simulink library "xpcueilib"  (Simulink 6.0)
settings: Solver=ode45  SolverMode=SingleTasking  StartTime=0.0  StopTime=10.0  RelTol=1e-3
(part 1 of 2)
settings Model: Creator=adowd  LastModifiedBy=adowd
settings DataIOCC: SignalLoggingName=logsOut
settings OptimizationCC: BooleanDataType=off
settings DebuggingCC: CheckExecutionContextPreStartOutputMsg=on  CheckExecutionContextRuntimeOutputMsg=on  SolverPrmCheckMsg=none
settings HardwareCC: TargetUnknown=on
settings GRTTargetCC: UtilityFuncGeneration=Automatic  LifeSpan=inf
settings SFSimCC: SFSimApplyToAllLibs=on  SFSimBuildMode=Incremental

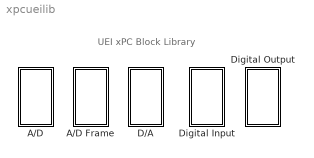
== system xpcueilib ==
  note: UEI xPC Block Library
  A/D : Subsystem  EnableExecutionContextPropagation=on
  A/D Frame : Subsystem  EnableExecutionContextPropagation=on
  D/A : Subsystem  EnableExecutionContextPropagation=on
  Digital Input : Subsystem  EnableExecutionContextPropagation=on
  Digital Output : Subsystem  EnableExecutionContextPropagation=on

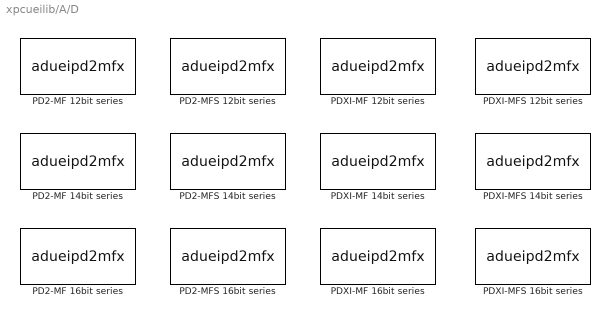
== system xpcueilib/A/D ==
  "PD2-MF 12bit series " : S-Function  InitFcn=muei  FunctionName=adueipd2mfx  Parameters=channel, gain, mux, range, sampletime, pcislot, boardType, gainval, board, devName  mask(ueipd2mf12_ad_7){boardtypein=PD2-MF-16-1M/12L, channel=[1], gain=[1], mux=[1], range=+- 10 Volts, sampletime=0.001, pcislot=-1}
      mask prompts: boardtypein "Board type:"; channel "Channel vector:"; gain "Gain vector:"; mux "Mux settling time vector (slow bit):"; pcislot "PCI slot (-1: autosearch):"
      mask help:
      | PD2-MF 12bit series
      | United Electronic Industries
      | Analog Input
      mask init:
      | [board, boardType, devName, gain, gainval, mux, maskdisplay, maskdescription]= madueipd2mfx(boardtypein,channel, gain, mux, pcislot);
      | set_param(gcb,'MaskDescription',maskdescription);
      | set_param(gcb,'MaskDisplay',maskdisplay);
      mask Help: helpview(fullfile(docroot, 'mapfiles', 'xpc.map'), 'UEI_PD2-MF-12bit-series_AD')
      mask StyleString: popup(PD2-MF-16-1M/12L|PD2-MF-16-1M/12H|PD2-MF-64-1M/12L|PD2-MF-64-1M/12H),edit,edit,edit,popup(+- 10 Volts|+- 5 Volts|0-10 Volts|0-5 Volts),edit,edit
      mask Display: disp('PD2-MF-16-1M/12L\nUEI\nAnalog Input');port_label('output',1,'1');
  "PD2-MF 14bit series " : S-Function  InitFcn=muei  FunctionName=adueipd2mfx  Parameters=channel, gain, mux, range, sampletime, pcislot, boardType, gainval, board, devName  mask(ueipd2mf14_ad_7){boardtypein=PD2-MF-16-400/14L, channel=[1], gain=[1], mux=[1], range=+- 10 Volts, sampletime=0.001, pcislot=-1}
      mask prompts: boardtypein "Board type:"; channel "Channel vector:"; gain "Gain vector:"; mux "Mux settling time vector (slow bit):"; pcislot "PCI slot (-1: autosearch):"
      mask help:
      | PD2-MF 14bit series
      | United Electronic Industries
      | Analog Input
      mask init: same as xpcueilib/A/D/PD2-MF 12bit series 
      mask Help: helpview(fullfile(docroot, 'mapfiles', 'xpc.map'), 'UEI_PD2-MF-14bit-series_AD')
      mask StyleString: popup(PD2-MF-16-400/14L|PD2-MF-16-400/14H|PD2-MF-64-400/14L|PD2-MF-64-400/14H|PD2-MF-16-800/14L|PD2-MF-16-800/14H|PD2-MF-64-800/14L|PD2-MF-64-800/14H|PD2-MF-16-2M/14L|PD2-MF-16-2M/14H|PD2-MF-64-2M/14L|PD2-MF-64-2M/14H),edit,edit,edit,popup(+- 10 Volts|+- 5 Volts|0-10 Volts|0-5 Volts),edit,edit
      mask Display: disp('PD2-MF-16-400/14L\nUEI\nAnalog Input');port_label('output',1,'1');
  "PD2-MF 16bit series " : S-Function  InitFcn=muei  FunctionName=adueipd2mfx  Parameters=channel, gain, mux, range, sampletime, pcislot, boardType, gainval, board, devName  mask(ueipd2mf16_ad_7){boardtypein=PD2-MF-16-333/16H, channel=[1], gain=[1], mux=[1], range=+- 10 Volts, sampletime=0.001, pcislot=-1}
      mask prompts: boardtypein "Board type:"; channel "Channel vector:"; gain "Gain vector:"; mux "Mux settling time vector (slow bit):"; pcislot "PCI slot (-1: autosearch):"
      mask help:
      | PD2-MF 16bit series
      | United Electronic Industries
      | Analog Input
      mask init: same as xpcueilib/A/D/PD2-MF 12bit series 
      mask Help: helpview(fullfile(docroot, 'mapfiles', 'xpc.map'), 'UEI_PD2-MF-16bit-series_AD')
      mask StyleString: popup(PD2-MF-16-50/16L|PD2-MF-16-50/16H|PD2-MF-64-50/16L|PD2-MF-64-50/16H|PD2-MF-16-150/16L|PD2-MF-16-150/16H|PD2-MF-64-150/16L|PD2-MF-64-150/16H|PD2-MF-16-333/16L|PD2-MF-16-333/16H|PD2-MF-64-333/16L|PD2-MF-64-333/16H|PD2-MF-16-500/16L|PD2-MF-16-500/16H|PD2-MF-64-500/16L|PD2-MF-64-500/16H),edit,edit,edit,popup(+- 10 Volts|+- 5 Volts|0-10 Volts|0-5 Volts),edit,edit
      mask Display: disp('PD2-MF-16-333/16H\nUEI\nAnalog Input');port_label('output',1,'1');
  "PD2-MFS 12bit series " : S-Function  InitFcn=muei  FunctionName=adueipd2mfx  Parameters=channel, gain, mux, range, sampletime, pcislot, boardType, gainval, board, devName  mask(ueipd2mfs12_ad_7){boardtypein=PD2-MFS-4-1M/12, channel=[1], gain=[1], mux=[1], range=+- 10 Volts, sampletime=0.001, pcislot=-1}
      mask prompts: boardtypein "Board type:"; channel "Channel vector:"; gain "Gain vector:"; mux "Mux settling time vector (slow bit):"; pcislot "PCI slot (-1: autosearch):"
      mask help:
      | PD2-MFS 12bit series
      | United Electronic Industries
      | Analog Input
      mask init: same as xpcueilib/A/D/PD2-MF 12bit series 
      mask Help: helpview(fullfile(docroot, 'mapfiles', 'xpc.map'), 'UEI_PD2-MFS-12bit-series_AD')
      mask StyleString: popup(PD2-MFS-4-1M/12|PD2-MFS-4-1M/12DG|PD2-MFS-4-1M/12H|PD2-MFS-8-1M/12|PD2-MFS-8-1M/12DG|PD2-MFS-8-1M/12H),edit,edit,edit,popup(+- 10 Volts|+- 5 Volts|0-10 Volts|0-5 Volts),edit,edit
      mask Display: disp('PD2-MFS-4-1M/12\nUEI\nAnalog Input');port_label('output',1,'1');
  "PD2-MFS 14bit series " : S-Function  InitFcn=muei  FunctionName=adueipd2mfx  Parameters=channel, gain, mux, range, sampletime, pcislot, boardType, gainval, board, devName  mask(ueipd2mfs14_ad_7){boardtypein=PD2-MFS-4-500/14, channel=[1], gain=[1], mux=[1], range=+- 10 Volts, sampletime=0.001, pcislot=-1}
      mask prompts: boardtypein "Board type:"; channel "Channel vector:"; gain "Gain vector:"; mux "Mux settling time vector (slow bit):"; pcislot "PCI slot (-1: autosearch):"
      mask help:
      | PD2-MFS 14bit series
      | United Electronic Industries
      | Analog Input
      mask init: same as xpcueilib/A/D/PD2-MF 12bit series 
      mask Help: helpview(fullfile(docroot, 'mapfiles', 'xpc.map'), 'UEI_PD2-MFS-14bit-series_AD')
      mask StyleString: popup(PD2-MFS-4-500/14|PD2-MFS-4-500/14DG|PD2-MFS-4-500/14H|PD2-MFS-8-500/14|PD2-MFS-8-500/14DG|PD2-MFS-8-500/14H|PD2-MFS-4-800/14|PD2-MFS-4-800/14DG|PD2-MFS-4-800/14H|PD2-MFS-8-800/14|PD2-MFS-8-800/14DG|PD2-MFS-8-800/14H|PD2-MFS-4-2M/14|PD2-MFS-4-2M/14DG|PD2-MFS-4-2M/14H|PD2-MFS-8-2M/14|PD2-MFS-8-2M/14DG|PD2-MFS-8-2M/14H),edit,edit,edit,popup(+- 10 Volts|+- 5 Volts|0-10 Volts|0-5 Volts),edit,edit
      mask Display: disp('PD2-MFS-4-500/14\nUEI\nAnalog Input');port_label('output',1,'1');
  "PD2-MFS 16bit series " : S-Function  InitFcn=muei  FunctionName=adueipd2mfx  Parameters=channel, gain, mux, range, sampletime, pcislot, boardType, gainval, board, devName  mask(ueipd2mfs16_ad_7){boardtypein=PD2-MFS-4-300/16, channel=[1], gain=[1], mux=[1], range=+- 10 Volts, sampletime=0.001, pcislot=-1}
      mask prompts: boardtypein "Board type:"; channel "Channel vector:"; gain "Gain vector:"; mux "Mux settling time vector (slow bit):"; pcislot "PCI slot (-1: autosearch):"
      mask help:
      | PD2-MFS 16bit series
      | United Electronic Industries
      | Analog Input
      mask init: same as xpcueilib/A/D/PD2-MF 12bit series 
      mask Help: helpview(fullfile(docroot, 'mapfiles', 'xpc.map'), 'UEI_PD2-MFS-16bit-series_AD')
      mask StyleString: popup(PD2-MFS-4-300/16|PD2-MFS-4-300/16DG|PD2-MFS-4-300/16H|PD2-MFS-8-300/16|PD2-MFS-8-300/16DG|PD2-MFS-8-300/16H|PD2-MFS-4-500/16|PD2-MFS-4-500/16DG|PD2-MFS-4-500/16H|PD2-MFS-8-500/16|PD2-MFS-8-500/16DG|PD2-MFS-8-500/16H),edit,edit,edit,popup(+- 10 Volts|+- 5 Volts|0-10 Volts|0-5 Volts),edit,edit
      mask Display: disp('PD2-MFS-4-300/16\nUEI\nAnalog Input');port_label('output',1,'1');
  "PDXI-MF 12bit series " : S-Function  InitFcn=muei  FunctionName=adueipd2mfx  Parameters=channel, gain, mux, range, sampletime, pcislot, boardType, gainval, board, devName  mask(ueipdximf12_ad_7){boardtypein=PDXI-MF-16-1M/12L, channel=[1], gain=[1], mux=[1], range=+- 10 Volts, sampletime=0.001, pcislot=-1}
      mask prompts: boardtypein "Board type:"; channel "Channel vector:"; gain "Gain vector:"; mux "Mux settling time vector (slow bit):"; pcislot "PCI slot (-1: autosearch):"
      mask help:
      | PDXI-MF 12bit series
      | United Electronic Industries
      | Analog Input
      mask init: same as xpcueilib/A/D/PD2-MF 12bit series 
      mask Help: helpview(fullfile(docroot, 'mapfiles', 'xpc.map'), 'UEI_PDXI-MF-12bit-series_AD')
      mask StyleString: popup(PDXI-MF-16-1M/12L|PDXI-MF-16-1M/12H|PDXI-MF-64-1M/12L|PDXI-MF-64-1M/12H),edit,edit,edit,popup(+- 10 Volts|+- 5 Volts|0-10 Volts|0-5 Volts),edit,edit
      mask Display: disp('PDXI-MF-16-1M/12L\nUEI\nAnalog Input');port_label('output',1,'1');
  "PDXI-MF 14bit series " : S-Function  InitFcn=muei  FunctionName=adueipd2mfx  Parameters=channel, gain, mux, range, sampletime, pcislot, boardType, gainval, board, devName  mask(ueipdximf14_ad_7){boardtypein=PDXI-MF-16-400/14L, channel=[1], gain=[1], mux=[1], range=+- 10 Volts, sampletime=0.001, pcislot=-1}
      mask prompts: boardtypein "Board type:"; channel "Channel vector:"; gain "Gain vector:"; mux "Mux settling time vector (slow bit):"; pcislot "PCI slot (-1: autosearch):"
      mask help:
      | PDXI-MF 14bit series
      | United Electronic Industries
      | Analog Input
      mask init: same as xpcueilib/A/D/PD2-MF 12bit series 
      mask Help: helpview(fullfile(docroot, 'mapfiles', 'xpc.map'), 'UEI_PDXI-MF-14bit-series_AD')
      mask StyleString: popup(PDXI-MF-16-400/14L|PDXI-MF-16-400/14H|PDXI-MF-64-400/14L|PDXI-MF-64-400/14H|PDXI-MF-16-800/14L|PDXI-MF-16-800/14H|PDXI-MF-64-800/14L|PDXI-MF-64-800/14H|PDXI-MF-16-2M/14L|PDXI-MF-16-2M/14H|PDXI-MF-64-2M/14L|PDXI-MF-64-2M/14H),edit,edit,edit,popup(+- 10 Volts|+- 5 Volts|0-10 Volts|0-5 Volts),edit,edit
      mask Display: disp('PDXI-MF-16-400/14L\nUEI\nAnalog Input');port_label('output',1,'1');
  "PDXI-MF 16bit series " : S-Function  InitFcn=muei  FunctionName=adueipd2mfx  Parameters=channel, gain, mux, range, sampletime, pcislot, boardType, gainval, board, devName  mask(ueipdximf16_ad_7){boardtypein=PDXI-MF-16-333/16H, channel=[1], gain=[1], mux=[1], range=+- 10 Volts, sampletime=0.001, pcislot=-1}
      mask prompts: boardtypein "Board type:"; channel "Channel vector:"; gain "Gain vector:"; mux "Mux settling time vector (slow bit):"; pcislot "PCI slot (-1: autosearch):"
      mask help:
      | PDXI-MF 16bit series
      | United Electronic Industries
      | Analog Input
      mask init: same as xpcueilib/A/D/PD2-MF 12bit series 
      mask Help: helpview(fullfile(docroot, 'mapfiles', 'xpc.map'), 'UEI_PDXI-MF-16bit-series_AD')
      mask StyleString: popup(PDXI-MF-16-50/16L|PDXI-MF-16-50/16H|PDXI-MF-64-50/16L|PDXI-MF-64-50/16H|PDXI-MF-16-150/16L|PDXI-MF-16-150/16H|PDXI-MF-64-150/16L|PDXI-MF-64-150/16H|PDXI-MF-16-333/16L|PDXI-MF-16-333/16H|PDXI-MF-64-333/16L|PDXI-MF-64-333/16H|PDXI-MF-16-500/16L|PDXI-MF-16-500/16H|PDXI-MF-64-500/16L|PDXI-MF-64-500/16H),edit,edit,edit,popup(+- 10 Volts|+- 5 Volts|0-10 Volts|0-5 Volts),edit,edit
      mask Display: disp('PDXI-MF-16-333/16H\nUEI\nAnalog Input');port_label('output',1,'1');
  "PDXI-MFS 12bit series " : S-Function  InitFcn=muei  FunctionName=adueipd2mfx  Parameters=channel, gain, mux, range, sampletime, pcislot, boardType, gainval, board, devName  mask(ueipd2mfs12_ad_7){boardtypein=PDXI-MFS-4-1M/12, channel=[1], gain=[1], mux=[1], range=+- 10 Volts, sampletime=0.001, pcislot=-1}
      mask prompts: boardtypein "Board type:"; channel "Channel vector:"; gain "Gain vector:"; mux "Mux settling time vector (slow bit):"; pcislot "PCI slot (-1: autosearch):"
      mask help:
      | PD2-MFS 12bit series
      | United Electronic Industries
      | Analog Input
      mask init: same as xpcueilib/A/D/PD2-MF 12bit series 
      mask Help: helpview(fullfile(docroot, 'mapfiles', 'xpc.map'), 'UEI_PDXI-MFS-12bit-series_AD')
      mask StyleString: popup(PDXI-MFS-4-1M/12|PDXI-MFS-4-1M/12DG|PDXI-MFS-4-1M/12H|PDXI-MFS-8-1M/12|PDXI-MFS-8-1M/12DG|PDXI-MFS-8-1M/12H),edit,edit,edit,popup(+- 10 Volts|+- 5 Volts|0-10 Volts|0-5 Volts),edit,edit
      mask Display: disp('PDXI-MFS-4-1M/12\nUEI\nAnalog Input');port_label('output',1,'1');
  "PDXI-MFS 14bit series " : S-Function  InitFcn=muei  FunctionName=adueipd2mfx  Parameters=channel, gain, mux, range, sampletime, pcislot, boardType, gainval, board, devName  mask(ueipd2mfs14_ad_7){boardtypein=PDXI-MFS-4-500/14, channel=[1], gain=[1], mux=[1], range=+- 10 Volts, sampletime=0.001, pcislot=-1}
      mask prompts: boardtypein "Board type:"; channel "Channel vector:"; gain "Gain vector:"; mux "Mux settling time vector (slow bit):"; pcislot "PCI slot (-1: autosearch):"
      mask help:
      | PD2-MFS 14bit series
      | United Electronic Industries
      | Analog Input
      mask init: same as xpcueilib/A/D/PD2-MF 12bit series 
      mask Help: helpview(fullfile(docroot, 'mapfiles', 'xpc.map'), 'UEI_PDXI-MFS-14bit-series_AD')
      mask StyleString: popup(PDXI-MFS-4-500/14|PDXI-MFS-4-500/14DG|PDXI-MFS-4-500/14H|PDXI-MFS-8-500/14|PDXI-MFS-8-500/14DG|PDXI-MFS-8-500/14H|PDXI-MFS-4-800/14|PDXI-MFS-4-800/14DG|PDXI-MFS-4-800/14H|PDXI-MFS-8-800/14|PDXI-MFS-8-800/14DG|PDXI-MFS-8-800/14H|PDXI-MFS-4-2M/14|PDXI-MFS-4-2M/14DG|PDXI-MFS-4-2M/14H|PDXI-MFS-8-2M/14|PDXI-MFS-8-2M/14DG|PDXI-MFS-8-2M/14H),edit,edit,edit,popup(+- 10 Volts|+- 5 Volts|0-10 Volts|0-5 Volts),edit,edit
      mask Display: disp('PDXI-MFS-4-500/14\nUEI\nAnalog Input');port_label('output',1,'1');
  "PDXI-MFS 16bit series " : S-Function  InitFcn=muei  FunctionName=adueipd2mfx  Parameters=channel, gain, mux, range, sampletime, pcislot, boardType, gainval, board, devName  mask(ueipd2mfs16_ad_7){boardtypein=PDXI-MFS-4-300/16, channel=[1], gain=[1], mux=[1], range=+- 10 Volts, sampletime=0.001, pcislot=-1}
      mask prompts: boardtypein "Board type:"; channel "Channel vector:"; gain "Gain vector:"; mux "Mux settling time vector (slow bit):"; pcislot "PCI slot (-1: autosearch):"
      mask help:
      | PD2-MFS 16bit series
      | United Electronic Industries
      | Analog Input
      mask init: same as xpcueilib/A/D/PD2-MF 12bit series 
      mask Help: helpview(fullfile(docroot, 'mapfiles', 'xpc.map'), 'UEI_PDXI-MFS-16bit-series_AD')
      mask StyleString: popup(PDXI-MFS-4-300/16|PDXI-MFS-4-300/16DG|PDXI-MFS-4-300/16H|PDXI-MFS-8-300/16|PDXI-MFS-8-300/16DG|PDXI-MFS-8-300/16H|PDXI-MFS-4-500/16|PDXI-MFS-4-500/16DG|PDXI-MFS-4-500/16H|PDXI-MFS-8-500/16|PDXI-MFS-8-500/16DG|PDXI-MFS-8-500/16H),edit,edit,edit,popup(+- 10 Volts|+- 5 Volts|0-10 Volts|0-5 Volts),edit,edit
      mask Display: disp('PDXI-MFS-4-300/16\nUEI\nAnalog Input');port_label('output',1,'1');

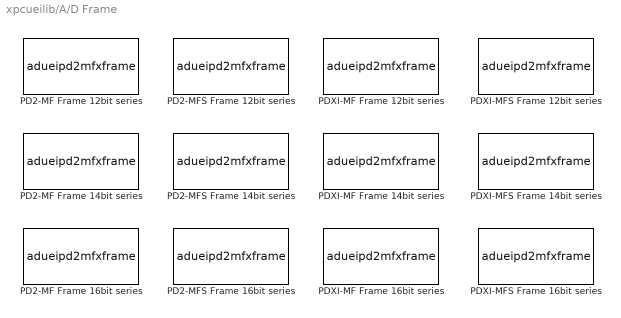
== system xpcueilib/A/D Frame ==
  "PD2-MF Frame 12bit series " : S-Function  InitFcn=muei  FunctionName=adueipd2mfxframe  Parameters=channel, gain, mux, range, sampletime, frametime, pcislot, boardType, gainval, board, devName, framesize, freq, sh, sediff, burst, nbursts, slave, outfmt, clsource  mask(ueipd2mf12_ad_16){boardtypein=PD2-MF-16-1M/12L, channel=[1], gain=[1], mux=[0], range=+- 10 Volts, sediff=Single Ended, framesize=32, outfmt=Frame (Signal Processing blockset needed), clsource=Internal, scantime=-1, frametime=0.001, sampletime=off, slave=off, freq=-1, burst=32, pcislot=-1}
      mask prompts: boardtypein "Board type:"; channel "Channel vector:"; gain "Gain vector:"; mux "Mux settling time vector (slow bit):"; sediff "Input coupling mode:"; framesize "Frame size:"; outfmt "Output format:"; clsource "Scan clock source:"; scantime "Scan time:"; frametime "Frame time:"; sampletime "Block is in an ISR:"; slave "Slave board:"; freq "Acquisition frequency:"; burst "DMA burst size:"; pcislot "PCI slot (-1: autosearch):"
      mask help:
      | PD2-MF 12bit series
      | United Electronic Industries
      | Analog Input
      mask init:
      | [board, boardType, devName, gain, gainval, mux, framesize, freq, frametime, scanfreq, sh, maskdisplay, maskdescription, burst, nbursts, sampletime]= madueipd2mfxframe(boardtypein,channel, gain, mux, framesize, freq, burst, scantime, sampletime, frametime, pcislot);
      | set_param(gcb,'MaskDescription',maskdescription);
      | set_param(gcb,'MaskDisplay',maskdisplay);
      mask Help: helpview(fullfile(docroot, 'mapfiles', 'xpc.map'), 'UEI_PD2-MF-12bit-Frame-series_AD')
      mask StyleString: popup(PD2-MF-16-1M/12L|PD2-MF-16-1M/12H|PD2-MF-64-1M/12L|PD2-MF-64-1M/12H),edit,edit,edit,popup(+- 10 Volts|+- 5 Volts|0-10 Volts|0-5 Volts),popup(Single Ended|Differential),edit,popup(Frame (Signal Processing blockset needed)|Vector),popup(Internal|External),edit,edit,checkbox,checkbox,edit,popup(32|16|8),edit
      mask Display: disp('PD2-MF-16-1M/12L\nUEI\nFrame Analog Input');port_label('output',1,'1');
  "PD2-MF Frame 14bit series " : S-Function  InitFcn=muei  FunctionName=adueipd2mfxframe  Parameters=channel, gain, mux, range, sampletime, frametime, pcislot, boardType, gainval, board, devName, framesize, freq, sh, sediff, burst, nbursts, slave, outfmt, clsource  mask(ueipd2mf14_ad_16){boardtypein=PD2-MF-16-400/14L, channel=[1], gain=[1], mux=[0], range=+- 10 Volts, sediff=Single Ended, framesize=32, outfmt=Frame (Signal Processing blockset needed), clsource=Internal, scantime=-1, frametime=0.001, sampletime=off, slave=off, freq=-1, burst=32, pcislot=-1}
      mask prompts: boardtypein "Board type:"; channel "Channel vector:"; gain "Gain vector:"; mux "Mux settling time vector (slow bit):"; sediff "Input coupling mode:"; framesize "Frame size:"; outfmt "Output format:"; clsource "Scan clock source:"; scantime "Scan time:"; frametime "Frame time:"; sampletime "Block is in an ISR"; slave "Slave board:"; freq "Acquisition frequency:"; burst "DMA burst size:"; pcislot "PCI slot (-1: autosearch):"
      mask help:
      | PD2-MF 14bit series
      | United Electronic Industries
      | Analog Input
      mask init:
      | [board, boardType, devName, gain, gainval, mux, framesize, freq, frametime, scanfreq, sh, maskdisplay, maskdescription, burst, nbursts, sampletime]= madueipd2mfxframe(boardtypein,channel, gain, mux, framesize, freq, burst, scantime, sampletime, frametime, pcislot);
      | set_param(gcb,'MaskDescription',maskdescription);
      | set_param(gcb,'MaskDisplay',maskdisplay);
      mask Help: helpview(fullfile(docroot, 'mapfiles', 'xpc.map'), 'UEI_PD2-MF-14bit-Frame-series_AD')
      mask StyleString: popup(PD2-MF-16-400/14L|PD2-MF-16-400/14H|PD2-MF-64-400/14L|PD2-MF-64-400/14H|PD2-MF-16-800/14L|PD2-MF-16-800/14H|PD2-MF-64-800/14L|PD2-MF-64-800/14H|PD2-MF-16-2M/14L|PD2-MF-16-2M/14H|PD2-MF-64-2M/14L|PD2-MF-64-2M/14H),edit,edit,edit,popup(+- 10 Volts|+- 5 Volts|0-10 Volts|0-5 Volts),popup(Single Ended|Differential),edit,popup(Frame (Signal Processing blockset needed)|Vector),popup(Internal|External),edit,edit,checkbox,checkbox,edit,popup(32|16|8),edit
      mask Display: disp('PD2-MF-16-400/14L\nUEI\nFrame Analog Input');port_label('output',1,'1');
  "PD2-MF Frame 16bit series " : S-Function  InitFcn=muei  FunctionName=adueipd2mfxframe  Parameters=channel, gain, mux, range, sampletime, frametime, pcislot, boardType, gainval, board, devName, framesize, freq, sh, sediff, burst, nbursts, slave, outfmt, clsource  mask(ueipd2mf16_ad_16){boardtypein=PD2-MF-16-333/16H, channel=[1], gain=[1], mux=[0], range=+- 10 Volts, sediff=Single Ended, framesize=32, outfmt=Frame (Signal Processing blockset needed), clsource=Internal, scantime=-1, frametime=0.001, sampletime=off, slave=off, freq=-1, burst=32, pcislot=-1}
      mask prompts: boardtypein "Board type:"; channel "Channel vector:"; gain "Gain vector:"; mux "Mux settling time vector (slow bit):"; sediff "Input coupling mode"; framesize "Frame size:"; outfmt "Output format:"; clsource "Scan clock source:"; scantime "Scan time:"; frametime "Frame time:"; sampletime "Block is in an ISR:"; slave "Slave board:"; freq "Acquisition frequency:"; burst "DMA burst size:"; pcislot "PCI slot (-1: autosearch):"
      mask help:
      | PD2-MF 16bit series
      | United Electronic Industries
      | Analog Input
      mask init:
      | [board, boardType, devName, gain, gainval, mux, framesize, freq, frametime, scanfreq, sh, maskdisplay, maskdescription, burst, nbursts, sampletime]= madueipd2mfxframe( boardtypein, channel, gain, mux, framesize, freq, burst, scantime, sampletime, frametime, pcislot );
      | set_param(gcb,'MaskDescription',maskdescription);
      | set_param(gcb,'MaskDisplay',maskdisplay);
      mask Help: helpview(fullfile(docroot, 'mapfiles', 'xpc.map'), 'UEI_PD2-MF-16bit-Frame-series_AD')
      mask StyleString: popup(PD2-MF-16-50/16L|PD2-MF-16-50/16H|PD2-MF-64-50/16L|PD2-MF-64-50/16H|PD2-MF-16-150/16L|PD2-MF-16-150/16H|PD2-MF-64-150/16L|PD2-MF-64-150/16H|PD2-MF-16-333/16L|PD2-MF-16-333/16H|PD2-MF-64-333/16L|PD2-MF-64-333/16H|PD2-MF-16-500/16L|PD2-MF-16-500/16H|PD2-MF-64-500/16L|PD2-MF-64-500/16H),edit,edit,edit,popup(+- 10 Volts|+- 5 Volts|0-10 Volts|0-5 Volts),popup(Single Ended|Differential),edit,popup(Frame (Signal Processing blockset needed)|Vector),popup(Internal|External),edit,edit,checkbox,checkbox,edit,popup(32|16|8),edit
      mask Display: disp('PD2-MF-16-333/16H\nUEI\nFrame Analog Input');port_label('output',1,'1');
  "PD2-MFS Frame 12bit series " : S-Function  InitFcn=muei  FunctionName=adueipd2mfxframe  Parameters=channel, gain, mux, range, sampletime, frametime, pcislot, boardType, gainval, board, devName, framesize, freq, sh, sediff, burst, nbursts, slave, outfmt, clsource  mask(ueipd2mfs12_ad_15){boardtypein=PD2-MFS-4-1M/12, channel=[1], gain=[1], mux=[0], range=+- 10 Volts, framesize=32, outfmt=Frame (Signal Processing blockset needed), clsource=Internal, scantime=-1, frametime=0.001, sampletime=off, slave=off, freq=-1, burst=32, pcislot=-1}
      mask prompts: boardtypein "Board type:"; channel "Channel vector:"; gain "Gain vector:"; mux "Mux settling time vector (slow bit):"; framesize "Frame size:"; outfmt "Output format:"; clsource "Scan clock source:"; scantime "Scan time:"; frametime "Frame time:"; sampletime "Block is in an ISR:"; slave "Slave board:"; freq "Acquisition frequency:"; burst "DMA burst size:"; pcislot "PCI slot (-1: autosearch):"
      mask help:
      | PD2-MFS 12bit series
      | United Electronic Industries
      | Analog Input
      mask init:
      | [board, boardType, devName, gain, gainval, mux, framesize, freq, frametime, scanfreq, sh, maskdisplay, maskdescription, burst, nbursts, sampletime]= madueipd2mfxframe(boardtypein,channel, gain, mux, framesize, freq, burst, scantime, sampletime, frametime, pcislot);
      | sediff = 1;
      | set_param(gcb,'MaskDescription',maskdescription);
      | set_param(gcb,'MaskDisplay',maskdisplay);
      mask Help: helpview(fullfile(docroot, 'mapfiles', 'xpc.map'), 'UEI_PD2-MFS-12bit-Frame-series_AD')
      mask StyleString: popup(PD2-MFS-4-1M/12|PD2-MFS-4-1M/12DG|PD2-MFS-4-1M/12H|PD2-MFS-8-1M/12|PD2-MFS-8-1M/12DG|PD2-MFS-8-1M/12H),edit,edit,edit,popup(+- 10 Volts|+- 5 Volts|0-10 Volts|0-5 Volts),edit,popup(Frame (Signal Processing blockset needed)|Vector),popup(Internal|External),edit,edit,checkbox,checkbox,edit,popup(32|16|8),edit
      mask Display: disp('PD2-MFS-4-1M/12\nUEI\nFrame Analog Input');port_label('output',1,'1');
  "PD2-MFS Frame 14bit series " : S-Function  InitFcn=muei  FunctionName=adueipd2mfxframe  Parameters=channel, gain, mux, range, sampletime, frametime, pcislot, boardType, gainval, board, devName, framesize, freq, sh, sediff, burst, nbursts, slave, outfmt, clsource  mask(ueipd2mfs14_ad_15){boardtypein=PD2-MFS-4-500/14, channel=[1], gain=[1], mux=[0], range=+- 10 Volts, framesize=32, outfmt=Frame (Signal Processing blockset needed), clsource=Internal, scantime=-1, frametime=0.001, sampletime=off, slave=off, freq=-1, burst=32, pcislot=-1}
      mask prompts: boardtypein "Board type:"; channel "Channel vector:"; gain "Gain vector:"; mux "Mux settling time vector (slow bit):"; framesize "Frame size:"; outfmt "Output format:"; clsource "Scan clock source:"; scantime "Scan time:"; frametime "Frame time:"; sampletime "Block is in an ISR:"; slave "Slave board:"; freq "Acquisition frequency"; burst "DMA burst size:"; pcislot "PCI slot (-1: autosearch):"
      mask help:
      | PD2-MFS 14bit series
      | United Electronic Industries
      | Analog Input
      mask init: same as xpcueilib/A/D Frame/PD2-MFS Frame 12bit series 
      mask Help: helpview(fullfile(docroot, 'mapfiles', 'xpc.map'), 'UEI_PD2-MFS-14bit-Frame-series_AD')
      mask StyleString: popup(PD2-MFS-4-500/14|PD2-MFS-4-500/14DG|PD2-MFS-4-500/14H|PD2-MFS-8-500/14|PD2-MFS-8-500/14DG|PD2-MFS-8-500/14H|PD2-MFS-4-800/14|PD2-MFS-4-800/14DG|PD2-MFS-4-800/14H|PD2-MFS-8-800/14|PD2-MFS-8-800/14DG|PD2-MFS-8-800/14H|PD2-MFS-4-2M/14|PD2-MFS-4-2M/14DG|PD2-MFS-4-2M/14H|PD2-MFS-8-2M/14|PD2-MFS-8-2M/14DG|PD2-MFS-8-2M/14H),edit,edit,edit,popup(+- 10 Volts|+- 5 Volts|0-10 Volts|0-5 Volts),edit,popup(Frame (Signal Processing blockset needed)|Vector),popup(Internal|External),edit,edit,checkbox,checkbox,edit,popup(32|16|8),edit
      mask Display: disp('PD2-MFS-4-500/14\nUEI\nFrame Analog Input');port_label('output',1,'1');
  "PD2-MFS Frame 16bit series " : S-Function  InitFcn=muei  FunctionName=adueipd2mfxframe  Parameters=channel, gain, mux, range, sampletime, frametime, pcislot, boardType, gainval, board, devName, framesize, freq, sh, sediff, burst, nbursts, slave, outfmt, clsource  mask(ueipd2mfs16_ad_15){boardtypein=PD2-MFS-4-300/16, channel=[1], gain=[1], mux=[0], range=+- 10 Volts, framesize=32, outfmt=Frame (Signal Processing blockset needed), clsource=Internal, scantime=-1, frametime=0.001, sampletime=off, slave=off, freq=-1, burst=32, pcislot=-1}
      mask prompts: boardtypein "Board type:"; channel "Channel vector:"; gain "Gain vector:"; mux "Mux settling time vector (slow bit):"; framesize "Frame size:"; outfmt "Output format:"; clsource "Scan clock source:"; scantime "Scan time:"; frametime "Frame time:"; sampletime "Block is in an ISR:"; slave "Slave board:"; freq "Acquisition frequency:"; burst "DMA burst size:"; pcislot "PCI slot (-1: autosearch):"
      mask help:
      | PD2-MFS 16bit series
      | United Electronic Industries
      | Analog Input
      mask init:
      | [board, boardType, devName, gain, gainval, mux, framesize, freq, frametime, scanfreq, sh, maskdisplay, maskdescription, burst, nbursts, sampletime]= madueipd2mfxframe(boardtypein,channel, gain, mux, framesize, freq, burst, scantime, sampletime, frametime, pcislot);
      | sediff = 1;
      | set_param(gcb,'MaskDescription',maskdescription);
      | set_param(gcb,'MaskDisplay',maskdisplay);
      mask Help: helpview(fullfile(docroot, 'mapfiles', 'xpc.map'), 'UEI_PD2-MFS-16bit-Frame-series_AD')
      mask StyleString: popup(PD2-MFS-4-300/16|PD2-MFS-4-300/16DG|PD2-MFS-4-300/16H|PD2-MFS-8-300/16|PD2-MFS-8-300/16DG|PD2-MFS-8-300/16H|PD2-MFS-4-500/16|PD2-MFS-4-500/16DG|PD2-MFS-4-500/16H|PD2-MFS-8-500/16|PD2-MFS-8-500/16DG|PD2-MFS-8-500/16H),edit,edit,edit,popup(+- 10 Volts|+- 5 Volts|0-10 Volts|0-5 Volts),edit,popup(Frame (Signal Processing blockset needed)|Vector),popup(Internal|External),edit,edit,checkbox,checkbox,edit,popup(32|16|8),edit
      mask Display: disp('PD2-MFS-4-300/16\nUEI\nFrame Analog Input');port_label('output',1,'1');
  "PDXI-MF Frame 12bit series " : S-Function  InitFcn=muei  FunctionName=adueipd2mfxframe  Parameters=channel, gain, mux, range, sampletime, frametime, pcislot, boardType, gainval, board, devName, framesize, freq, sh, sediff, burst, nbursts, slave, outfmt, clsource  mask(ueipdximf12_ad_16){boardtypein=PDXI-MF-16-1M/12L, channel=[1], gain=[1], mux=[0], range=+- 10 Volts, sediff=Single Ended, framesize=32, outfmt=Frame (Signal Processing blockset needed), clsource=Internal, scantime=-1, frametime=0.001, sampletime=off, slave=off, freq=-1, burst=32, pcislot=-1}
      mask prompts: boardtypein "Board type:"; channel "Channel vector:"; gain "Gain vector:"; mux "Mux settling time vector (slow bit):"; sediff "Input coupling mode:"; framesize "Frame size:"; outfmt "Output format:"; clsource "Scan clock source:"; scantime "Scan time:"; frametime "Frame time:"; sampletime "Block is in an ISR:"; slave "Slave board:"; freq "Acquisition frequency:"; burst "DMA burst size:"; pcislot "PCI slot (-1: autosearch):"
      mask help:
      | PDXI-MF 12bit series
      | United Electronic Industries
      | Analog Input
      mask init: same as xpcueilib/A/D Frame/PD2-MF Frame 12bit series 
      mask Help: helpview(fullfile(docroot, 'mapfiles', 'xpc.map'), 'UEI_PDXI-MF-12bit-Frame-series_AD')
      mask StyleString: popup(PDXI-MF-16-1M/12L|PDXI-MF-16-1M/12H|PDXI-MF-64-1M/12L|PDXI-MF-64-1M/12H),edit,edit,edit,popup(+- 10 Volts|+- 5 Volts|0-10 Volts|0-5 Volts),popup(Single Ended|Differential),edit,popup(Frame (Signal Processing blockset needed)|Vector),popup(Internal|External),edit,edit,checkbox,checkbox,edit,popup(32|16|8),edit
      mask Display: disp('PDXI-MF-16-1M/12L\nUEI\nFrame Analog Input');port_label('output',1,'1');
  "PDXI-MF Frame 14bit series " : S-Function  InitFcn=muei  FunctionName=adueipd2mfxframe  Parameters=channel, gain, mux, range, sampletime, frametime, pcislot, boardType, gainval, board, devName, framesize, freq, sh, sediff, burst, nbursts, slave, outfmt, clsource  mask(ueipdximf14_ad_16){boardtypein=PDXI-MF-16-400/14L, channel=[1], gain=[1], mux=[0], range=+- 10 Volts, sediff=Single Ended, framesize=32, outfmt=Frame (Signal Processing blockset needed), clsource=Internal, scantime=-1, frametime=0.001, sampletime=off, slave=off, freq=-1, burst=32, pcislot=-1}
      mask prompts: boardtypein "Board type:"; channel "Channel vector:"; gain "Gain vector:"; mux "Mux settling time vector (slow bit):"; sediff "Input coupling mode:"; framesize "Frame size:"; outfmt "Output format:"; clsource "Scan clock source:"; scantime "Scan time:"; frametime "Frame time:"; sampletime "Block is in an ISR"; slave "Slave board:"; freq "Acquisition frequency:"; burst "DMA burst size:"; pcislot "PCI slot (-1: autosearch):"
      mask help:
      | PDXI-MF 14bit series
      | United Electronic Industries
      | Analog Input
      mask init: same as xpcueilib/A/D Frame/PD2-MF Frame 14bit series 
      mask Help: helpview(fullfile(docroot, 'mapfiles', 'xpc.map'), 'UEI_PDXI-MF-14bit-Frame-series_AD')
      mask StyleString: popup(PDXI-MF-16-400/14L|PDXI-MF-16-400/14H|PDXI-MF-64-400/14L|PDXI-MF-64-400/14H|PDXI-MF-16-800/14L|PDXI-MF-16-800/14H|PDXI-MF-64-800/14L|PDXI-MF-64-800/14H|PDXI-MF-16-2M/14L|PDXI-MF-16-2M/14H|PDXI-MF-64-2M/14L|PDXI-MF-64-2M/14H),edit,edit,edit,popup(+- 10 Volts|+- 5 Volts|0-10 Volts|0-5 Volts),popup(Single Ended|Differential),edit,popup(Frame (Signal Processing blockset needed)|Vector),popup(Internal|External),edit,edit,checkbox,checkbox,edit,popup(32|16|8),edit
      mask Display: disp('PDXI-MF-16-400/14L\nUEI\nFrame Analog Input');port_label('output',1,'1');
  "PDXI-MF Frame 16bit series " : S-Function  InitFcn=muei  FunctionName=adueipd2mfxframe  Parameters=channel, gain, mux, range, sampletime, frametime, pcislot, boardType, gainval, board, devName, framesize, freq, sh, sediff, burst, nbursts, slave, outfmt, clsource  mask(ueipdximf16_ad_16){boardtypein=PDXI-MF-16-333/16H, channel=[1], gain=[1], mux=[0], range=+- 10 Volts, sediff=Single Ended, framesize=32, outfmt=Frame (Signal Processing blockset needed), clsource=Internal, scantime=-1, frametime=0.001, sampletime=off, slave=off, freq=-1, burst=32, pcislot=-1}
      mask prompts: boardtypein "Board type:"; channel "Channel vector:"; gain "Gain vector:"; mux "Mux settling time vector (slow bit):"; sediff "Input coupling mode"; framesize "Frame size:"; outfmt "Output format:"; clsource "Scan clock source:"; scantime "Scan time:"; frametime "Frame time:"; sampletime "Block is in an ISR:"; slave "Slave board:"; freq "Acquisition frequency:"; burst "DMA burst size:"; pcislot "PCI slot (-1: autosearch):"
      mask help:
      | PDXI-MF 16bit series
      | United Electronic Industries
      | Analog Input
      mask init: same as xpcueilib/A/D Frame/PD2-MF Frame 16bit series 
      mask Help: helpview(fullfile(docroot, 'mapfiles', 'xpc.map'), 'UEI_PDXI-MF-16bit-Frame-series_AD')
      mask StyleString: popup(PDXI-MF-16-50/16L|PDXI-MF-16-50/16H|PDXI-MF-64-50/16L|PDXI-MF-64-50/16H|PDXI-MF-16-150/16L|PDXI-MF-16-150/16H|PDXI-MF-64-150/16L|PDXI-MF-64-150/16H|PDXI-MF-16-333/16L|PDXI-MF-16-333/16H|PDXI-MF-64-333/16L|PDXI-MF-64-333/16H|PDXI-MF-16-500/16L|PDXI-MF-16-500/16H|PDXI-MF-64-500/16L|PDXI-MF-64-500/16H),edit,edit,edit,popup(+- 10 Volts|+- 5 Volts|0-10 Volts|0-5 Volts),popup(Single Ended|Differential),edit,popup(Frame (Signal Processing blockset needed)|Vector),popup(Internal|External),edit,edit,checkbox,checkbox,edit,popup(32|16|8),edit
      mask Display: disp('PDXI-MF-16-333/16H\nUEI\nFrame Analog Input');port_label('output',1,'1');
  "PDXI-MFS Frame 12bit series " : S-Function  InitFcn=muei  FunctionName=adueipd2mfxframe  Parameters=channel, gain, mux, range, sampletime, frametime, pcislot, boardType, gainval, board, devName, framesize, freq, sh, sediff, burst, nbursts, slave, outfmt, clsource  mask(ueipdximfs12_ad_15){boardtypein=PDXI-MFS-4-1M/12, channel=[1], gain=[1], mux=[0], range=+- 10 Volts, framesize=32, outfmt=Frame (Signal Processing blockset needed), clsource=Internal, scantime=-1, frametime=0.001, sampletime=off, slave=off, freq=-1, burst=32, pcislot=-1}
      mask prompts: boardtypein "Board type:"; channel "Channel vector:"; gain "Gain vector:"; mux "Mux settling time vector (slow bit):"; framesize "Frame size:"; outfmt "Output format:"; clsource "Scan clock source:"; scantime "Scan time:"; frametime "Frame time:"; sampletime "Block is in an ISR:"; slave "Slave board:"; freq "Acquisition frequency:"; burst "DMA burst size:"; pcislot "PCI slot (-1: autosearch):"
      mask help:
      | PDXI-MFS 12bit series
      | United Electronic Industries
      | Analog Input
      mask init: same as xpcueilib/A/D Frame/PD2-MFS Frame 12bit series 
      mask Help: helpview(fullfile(docroot, 'mapfiles', 'xpc.map'), 'UEI_PDXI-MFS-12bit-Frame-series_AD')
      mask StyleString: popup(PDXI-MFS-4-1M/12|PDXI-MFS-4-1M/12DG|PDXI-MFS-4-1M/12H|PDXI-MFS-8-1M/12|PDXI-MFS-8-1M/12DG|PDXI-MFS-8-1M/12H),edit,edit,edit,popup(+- 10 Volts|+- 5 Volts|0-10 Volts|0-5 Volts),edit,popup(Frame (Signal Processing blockset needed)|Vector),popup(Internal|External),edit,edit,checkbox,checkbox,edit,popup(32|16|8),edit
      mask Display: disp('PDXI-MFS-4-1M/12\nUEI\nFrame Analog Input');port_label('output',1,'1');
  "PDXI-MFS Frame 14bit series " : S-Function  InitFcn=muei  FunctionName=adueipd2mfxframe  Parameters=channel, gain, mux, range, sampletime, frametime, pcislot, boardType, gainval, board, devName, framesize, freq, sh, sediff, burst, nbursts, slave, outfmt, clsource  mask(ueipdximfs14_ad_15){boardtypein=PDXI-MFS-4-500/14, channel=[1], gain=[1], mux=[0], range=+- 10 Volts, framesize=32, outfmt=Frame (Signal Processing blockset needed), clsource=Internal, scantime=-1, frametime=0.001, sampletime=off, slave=off, freq=-1, burst=32, pcislot=-1}
      mask prompts: boardtypein "Board type:"; channel "Channel vector:"; gain "Gain vector:"; mux "Mux settling time vector (slow bit):"; framesize "Frame size:"; outfmt "Output format:"; clsource "Scan clock source:"; scantime "Scan time:"; frametime "Frame time:"; sampletime "Block is in an ISR:"; slave "Slave board:"; freq "Acquisition frequency"; burst "DMA burst size:"; pcislot "PCI slot (-1: autosearch):"
      mask help:
      | PDXI-MFS 14bit series
      | United Electronic Industries
      | Analog Input
      mask init: same as xpcueilib/A/D Frame/PD2-MFS Frame 12bit series 
      mask Help: helpview(fullfile(docroot, 'mapfiles', 'xpc.map'), 'UEI_PDXI-MFS-14bit-Frame-series_AD')
      mask StyleString: popup(PDXI-MFS-4-500/14|PDXI-MFS-4-500/14DG|PDXI-MFS-4-500/14H|PDXI-MFS-8-500/14|PDXI-MFS-8-500/14DG|PDXI-MFS-8-500/14H|PDXI-MFS-4-800/14|PDXI-MFS-4-800/14DG|PDXI-MFS-4-800/14H|PDXI-MFS-8-800/14|PDXI-MFS-8-800/14DG|PDXI-MFS-8-800/14H|PDXI-MFS-4-2M/14|PDXI-MFS-4-2M/14DG|PDXI-MFS-4-2M/14H|PDXI-MFS-8-2M/14|PDXI-MFS-8-2M/14DG|PDXI-MFS-8-2M/14H),edit,edit,edit,popup(+- 10 Volts|+- 5 Volts|0-10 Volts|0-5 Volts),edit,popup(Frame (Signal Processing blockset needed)|Vector),popup(Internal|External),edit,edit,checkbox,checkbox,edit,popup(32|16|8),edit
      mask Display: disp('PDXI-MFS-4-500/14\nUEI\nFrame Analog Input');port_label('output',1,'1');
  "PDXI-MFS Frame 16bit series " : S-Function  InitFcn=muei  FunctionName=adueipd2mfxframe  Parameters=channel, gain, mux, range, sampletime, frametime, pcislot, boardType, gainval, board, devName, framesize, freq, sh, sediff, burst, nbursts, slave, outfmt, clsource  mask(ueipdximfs16_ad_15){boardtypein=PDXI-MFS-4-300/16, channel=[1], gain=[1], mux=[0], range=+- 10 Volts, framesize=32, outfmt=Frame (Signal Processing blockset needed), clsource=Internal, scantime=-1, frametime=0.001, sampletime=off, slave=off, freq=-1, burst=32, pcislot=-1}
      mask prompts: boardtypein "Board type:"; channel "Channel vector:"; gain "Gain vector:"; mux "Mux settling time vector (slow bit):"; framesize "Frame size:"; outfmt "Output format:"; clsource "Scan clock source:"; scantime "Scan time:"; frametime "Frame time:"; sampletime "Block is in an ISR:"; slave "Slave board:"; freq "Acquisition frequency:"; burst "DMA burst size:"; pcislot "PCI slot (-1: autosearch):"
      mask help:
      | PDXI-MFS 16bit series
      | United Electronic Industries
      | Analog Input
      mask init: same as xpcueilib/A/D Frame/PD2-MFS Frame 16bit series 
      mask Help: helpview(fullfile(docroot, 'mapfiles', 'xpc.map'), 'UEI_PDXI-MFS-16bit-Frame-series_AD')
      mask StyleString: popup(PDXI-MFS-4-300/16|PDXI-MFS-4-300/16DG|PDXI-MFS-4-300/16H|PDXI-MFS-8-300/16|PDXI-MFS-8-300/16DG|PDXI-MFS-8-300/16H|PDXI-MFS-4-500/16|PDXI-MFS-4-500/16DG|PDXI-MFS-4-500/16H|PDXI-MFS-8-500/16|PDXI-MFS-8-500/16DG|PDXI-MFS-8-500/16H),edit,edit,edit,popup(+- 10 Volts|+- 5 Volts|0-10 Volts|0-5 Volts),edit,popup(Frame (Signal Processing blockset needed)|Vector),popup(Internal|External),edit,edit,checkbox,checkbox,edit,popup(32|16|8),edit
      mask Display: disp('PDXI-MFS-4-300/16\nUEI\nFrame Analog Input');port_label('output',1,'1');
